simulink model "simpleHelicopter_ROM"  (R2023b)
settings: Solver=FixedStepAuto  StartTime=0.0  StopTime=500  FixedStep=fixedStepSize  RelTol=1e-3
model workspace: external: MATLAB File .\turboShaftEngine\initialization.m (data not in the file)
libraries: fl_lib x3, simulink x2, nesl_utility x2, SignalEditorBlockLib x1, aerolibatmos2 x1
settings Model: Creator=imyrsini  LastModifiedBy=imyrsini
settings HardwareCC: ProdBitPerLong=64  ProdHWDeviceType=Intel->x86-64 (Linux 64)
settings RTWCC: Description=Simulink Desktop Real-Time  SystemTargetFile=sldrt.tlc  TemplateMakefile=sldrt.tmf  RTWCompilerOptimization=on
settings CodeAppCC: MaxIdLength=95
settings SimulinkDesktopRealTimeCC: TargetLibSuffix=_sldrt.a  TargetPreCompLibLocation=L:\ML_MATLAB64\R2023b\toolbox\sldrt\lib\win64

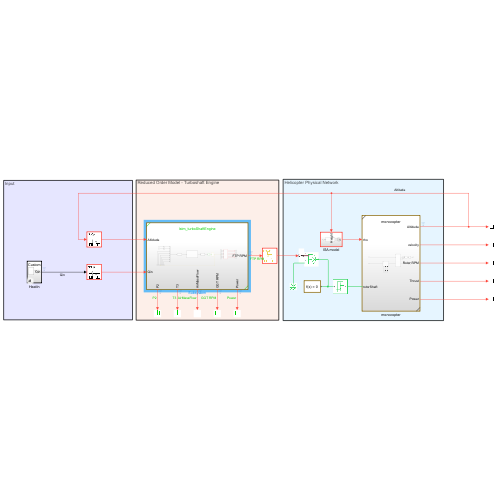
[thumbnail: Simulink's stored preview of the top-level diagram]
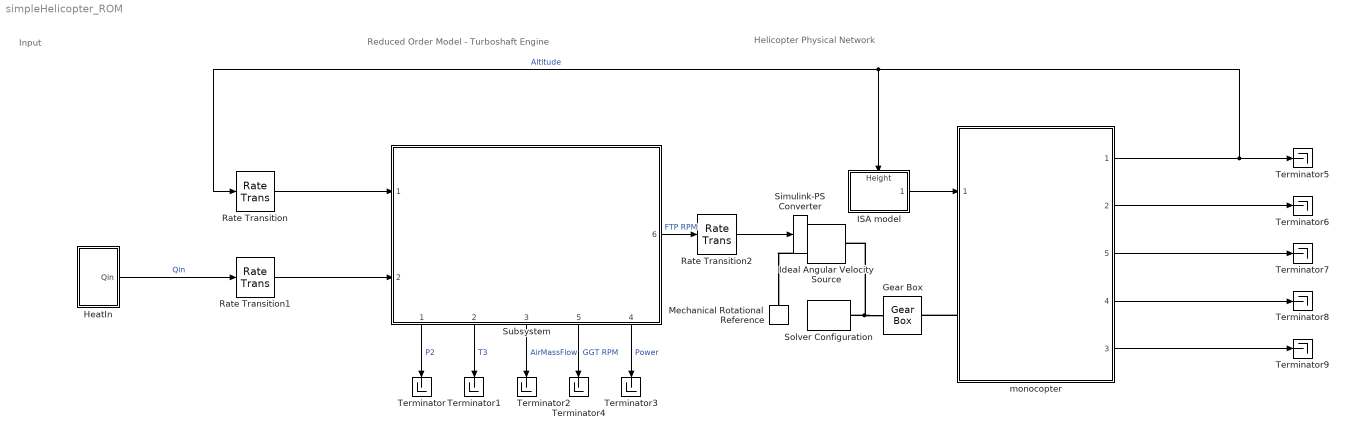
== system simpleHelicopter_ROM ==
  note: Helicopter Physical Network
  note: Reduced Order Model - Turboshaft Engine
  note: Input
  Gear Box : fl_lib/Mechanical/Mechanisms/Gear Box  ratio=shaftFTP.GearRatio  t_in_specify=off  t_in_priority=None  t_in=0 N*m  t_in_nominal_specify=off  t_in_nominal_unit=N*m  t_in_nominal_value=1  t_out_specify=off  t_out_priority=None  t_out=0 N*m  t_out_nominal_specify=off  t_out_nominal_unit=N*m  t_out_nominal_value=1
  HeatIn : Subsystem  Variant=on  VariantControlMode=label  VariantControl=Choice  LabelModeActiveChoice=Custom
  ISA model : Subsystem
      settings: PortSchema="{\"entries\":[{\"content\":{\"sides\":[{\"content\":{},\"type\":\"ConnectorPlacement.EquallySpacedRectSide\",\"uuid\":\"cd3fd5c5-2b63-41b8-986b-cb0626d922c8\"},{\"content\":{\"connectorIds\":[\"Out1\"],\"side\":\"RIGHT\"},\"type\":\"ConnectorPlacement.EquallySpacedRectSide\",\"uuid\":\"f88a6424-224e-4f39-ae1f-8f87a37f52da\"},{\"content\":{\"connectorIds\":[\"In1\"],\"side\":\"TOP\"},\"type\":\"ConnectorPlacement.EquallySpacedRectSide\",\"uuid\":\"a5abf431-3271-4a9a-98cd-2e875e4fe311\"}]},\"type\":\"ConnectorPlacement.EquallySpacedConnector\",\"uuid\":\"1dfe5bef-2257-4bff-bfbf-b68a279f2918\"}],\"packageUris\":[\"http://schema.mathworks.com/mf0/Connector/R2020b\"],\"version\":\"1.0\"}"
  Ideal Angular Velocity Source : fl_lib/Mechanical/Mechanical Sources/Ideal Angular Velocity Source
  Mechanical Rotational Reference : fl_lib/Mechanical/Rotational Elements/Mechanical Rotational Reference
  Rate Transition : RateTransition  Integrity=off  OutPortSampleTime=sampleTime
  Rate Transition1 : RateTransition  Integrity=off  OutPortSampleTime=sampleTime
  Rate Transition2 : RateTransition  OutPortSampleTime=sampleTime
  Simulink-PS Converter : nesl_utility/Simulink-PS Converter  PhysicalDomain=network_engine_domain  SubClassName=ps_input  LeftPortType=input  RightPortType=output  PseudoPeriodic=off  Frequencies=[]  NoiseDistribution=none  NoiseParameters=[]  Unit=rpm  AffineConversion=off  FilteringAndDerivatives=filter  SimscapeFilterOrder=2  InputFilterTimeConstant=fixedStepSize  UdotUserProvided=0
  Solver Configuration : nesl_utility/Solver Configuration  PhysicalDomain=network_engine_domain  SubClassName=solver  LeftPortType=input  RightPortType=generic  Tones=[]  Harmonics=[]  SimulateNoise=off  Profile=off  UseLocalSampling=off  EnableSwitchedLinearOptims=on  FrequencyDomain=off  UseCCode=off  RelTol=0.001  AbsTol=0.001  MinStep=1e-09  ToWorkspace=off  RevertToSquareIcSolve=off  NumHomotopyIterations=100  PhasorMode=off  PhasorModeNumHarmonics=1  ConsistencySolver=NEWTON_XTOL_AFTER_FTOL  IndexReductionMethod=DerivativeReplacement  DoDC=on  ResidualTolerance=1e-09  ConsistencyTolSource=GLOBAL  ConsistencyAbsTol=0.001  ConsistencyRelTol=0.001  ConsistencyTolFactor=0.001  UseLocalSolver=off  LocalSolverChoice=NE_BACKWARD_EULER_ADVANCER  ResolveIndetEquations=on  FunctionEvalNumThread=1  LocalSolverSampleTime=0.001  DoFixedCost=off  MaxNonlinIter=3  MaxModeIter=2  ComputeImpulses=off  ImpulseIterations=2  LinearAlgebra=auto  LinearAlgebraNumThread=0  EquationFormulation=NE_TIME_EF  DelaysMemoryBudget=1024  AutomaticFiltering=on  FilteringTimeConstant=0.001  PartitionStorageMethod=AS_NEEDED  PartitionMemoryBudget=1024  PartitionMethod=ROBUST  MultibodyUseLocalSolver=off  MultibodyLocalSolverChoice=ODE1  MultibodyLocalSolverSampleTime=0.001
  Subsystem : Subsystem  ReferencedSubsystem=lstm_turboShaftEngine
      settings: PortSchema="{\"entries\":[{\"content\":{\"sides\":[{\"content\":{\"connectorIds\":[\"In1\",\"In2\"]},\"type\":\"ConnectorPlacement.EquallySpacedRectSide\",\"uuid\":\"7920ffa2-fa35-490a-8d2a-d5dfbe6c6590\"},{\"content\":{\"connectorIds\":[\"Out6\"],\"side\":\"RIGHT\"},\"type\":\"ConnectorPlacement.EquallySpacedRectSide\",\"uuid\":\"83125dc3-a557-4488-80f1-9e314febf824\"},{\"content\":{\"side\":\"TOP\"},\"type\":\"ConnectorPlacement.EquallySpacedRectSide\",\"uuid\":\"ba262837-84ff-4985-9619-929dd124c29a\"},{\"content\":{\"connectorIds\":[\"Out1\",\"Out2\",\"Out3\",\"Out5\",\"Out4\"],\"side\":\"BOTTOM\"},\"type\":\"ConnectorPlacement.EquallySpacedRectSide\",\"uuid\":\"009c9890-7b19-4ffc-b0a7-3325114fea5d\"}]},\"type\":\"ConnectorPlacement.EquallySpacedConnector\",\"uuid\":\"400dc66e-59e5-4048-8df8-84772b11b1df\"}],\"packageUris\":[\"http://schema.mathworks.com/mf0/Connector/R2020b\"],\"version\":\"1.0\"}"
  Terminator{,1..9} (10 alike) : Terminator
  monocopter : Subsystem  ReferencedSubsystem=monocopter
      settings: PortSchema="{\"entries\":[{\"content\":{\"sides\":[{\"content\":{\"connectorIds\":[\"In1\",\"LConn1\"]},\"type\":\"ConnectorPlacement.EquallySpacedRectSide\",\"uuid\":\"2ecbf831-8a46-4c85-bf63-980a752dd5b1\"},{\"content\":{\"connectorIds\":[\"Out1\",\"Out2\",\"Out5\",\"Out4\",\"Out3\"],\"side\":\"RIGHT\"},\"type\":\"ConnectorPlacement.EquallySpacedRectSide\",\"uuid\":\"e1b9456e-2a06-4a0b-bd2d-ca850f525143\"},{\"content\":{\"side\":\"TOP\"},\"type\":\"ConnectorPlacement.EquallySpacedRectSide\",\"uuid\":\"495d5151-b094-4c59-ad95-48151a95ddaf\"},{\"content\":{\"side\":\"BOTTOM\"},\"type\":\"ConnectorPlacement.EquallySpacedRectSide\",\"uuid\":\"d711d358-7c2d-4243-addb-9f7f6c9821dd\"}]},\"type\":\"ConnectorPlacement.EquallySpacedConnector\",\"uuid\":\"3949e89b-de6d-4024-bd06-1eddfa87edaa\"}],\"packageUris\":[\"http://schema.mathworks.com/mf0/Connector/R2020b\"],\"version\":\"1.0\"}"
  wires:
  Rate Transition/1 -> Subsystem/1
  Rate Transition1/1 -> Subsystem/2
  Subsystem/6 -> Rate Transition2/1  "FTP RPM"
  Subsystem/1 -> Terminator/1  "P2"
  Subsystem/2 -> Terminator1/1  "T3"
  Subsystem/3 -> Terminator2/1  "AirMassFlow"
  Subsystem/4 -> Terminator3/1  "Power"
  Subsystem/5 -> Terminator4/1  "GGT RPM"
  Rate Transition2/1 -> Simulink-PS Converter/1
  monocopter/1 -> Terminator5/1, Rate Transition/1, ISA model/1(Height)  "Altitude"
  ISA model/1(Outport) -> monocopter/1
  monocopter/2 -> Terminator6/1
  monocopter/5 -> Terminator7/1
  monocopter/4 -> Terminator8/1
  monocopter/3 -> Terminator9/1
  HeatIn/1(Qin) -> Rate Transition1/1  "Qin"
  connections:
  Solver Configuration/RConn1 -- Ideal Angular Velocity Source/LConn1 -- Gear Box/LConn1
  Simulink-PS Converter/RConn1 -- Ideal Angular Velocity Source/RConn1
  Ideal Angular Velocity Source/RConn2 -- Mechanical Rotational Reference/LConn1
  monocopter/LConn1 -- Gear Box/RConn1

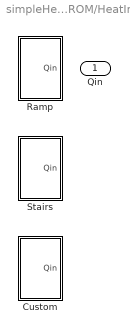
== system simpleHelicopter_ROM/HeatIn ==
  Custom : Subsystem  VariantControl=Custom
  Ramp : Subsystem  VariantControl=Ramp
  Stairs : Subsystem  VariantControl=Stairs
  Qin : Outport

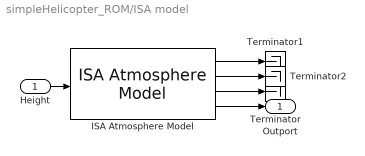
== system simpleHelicopter_ROM/ISA model ==
  Height : Inport
  ISA Atmosphere Model : aerolibatmos2/ISA Atmosphere Model  useExtended=off  action=Warning  custom=off  viscosityOut=off  g=9.80665  gamma=1.4  R=287.0531  L=0.0065  h_trop=11000  h_strat=20000  rho0=1.225  P0=101325  T0=288.15  h0=0
  Terminator : Terminator
  Terminator1 : Terminator
  Terminator2 : Terminator
  Outport : Outport
  wires:
  ISA Atmosphere Model/3 -> Terminator/1
  ISA Atmosphere Model/2 -> Terminator2/1
  Height/1 -> ISA Atmosphere Model/1
  ISA Atmosphere Model/1 -> Terminator1/1
  ISA Atmosphere Model/4 -> Outport/1

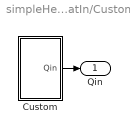
== system simpleHelicopter_ROM/HeatIn/Custom ==
  Custom : Subsystem  VariantControl=Custom
  Qin : Outport
  wires:
  Custom/1(Qin) -> Qin/1

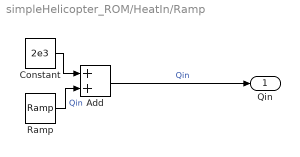
== system simpleHelicopter_ROM/HeatIn/Ramp ==
  Add : Sum
  Constant : Constant  Value=2e3
  Ramp : simulink/Sources/Ramp  slope=6  start=rom.init.timeColdStart  InitialOutput=0
  Qin : Outport
  wires:
  Ramp/1 -> Add/2  "Qin"
  Constant/1 -> Add/1
  Add/1 -> Qin/1  "Qin"

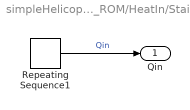
== system simpleHelicopter_ROM/HeatIn/Stairs ==
  Repeating Sequence1 : simulink/Sources/Repeating Sequence  rep_seq_t=Qin_time  rep_seq_y=Qin
  Qin : Outport
  wires:
  Repeating Sequence1/1 -> Qin/1  "Qin"

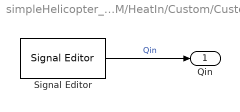
== system simpleHelicopter_ROM/HeatIn/Custom/Custom ==
  Signal Editor : SignalEditorBlockLib/Signal Editor  FileName=testScenario.mat  ActiveScenario=Scenario  ActiveSignal=Signal 1  IsBus=off  OutputBusObjectStr=Bus: BusObject  SampleTime=0  ZeroCross=off  OutputAfterFinalValue=Setting to zero  Unit=inherit  PreserveSignalName=on  ApplySigPropsToAllScenarios=on  ApplySigPropsToAllSignals=off
  Qin : Outport
  wires:
  Signal Editor/1 -> Qin/1  "Qin"
